simulink model "close_loop"  (R2018a)
settings: Solver=ode4  StartTime=0.0  StopTime=4  FixedStep=0.001  RelTol=1e-3
undefined symbols (not defined in the file): Kd, Ki, Km, Kp, Wm, Zm
settings Model: Creator=msi  LastModifiedBy=xde12

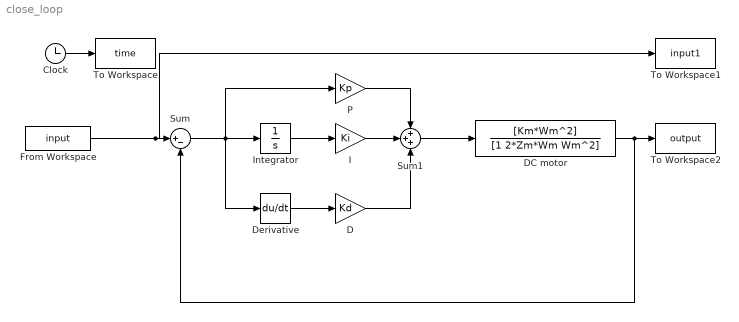
== system close_loop ==
  Clock : Clock
  D : Gain  Gain=Kd
  DC motor : TransferFcn  Numerator=[Km*Wm^2]  Denominator=[1 2*Zm*Wm Wm^2]
  Derivative : Derivative
  From Workspace : FromWorkspace  VariableName=input  SampleTime=0
  I : Gain  Gain=Ki
  Integrator : Integrator
  P : Gain  Gain=Kp
  Sum : Sum  Inputs=|+-
  Sum1 : Sum  Inputs=+++
  To Workspace : ToWorkspace  VariableName=time  SampleTime=-1
  To Workspace1 : ToWorkspace  VariableName=input1  SampleTime=-1
  To Workspace2 : ToWorkspace  VariableName=output  SampleTime=-1
  wires:
  Sum/1 -> Derivative/1, P/1, Integrator/1
  Integrator/1 -> I/1
  Derivative/1 -> D/1
  P/1 -> Sum1/1
  I/1 -> Sum1/2
  D/1 -> Sum1/3
  DC motor/1 -> To Workspace2/1, Sum/2
  Sum1/1 -> DC motor/1
  Clock/1 -> To Workspace/1
  From Workspace/1 -> To Workspace1/1, Sum/1
